simulink model "Main_detection"  (R2015a)
settings: Solver=ode3  StartTime=0.0  StopTime=15  RelTol=1e-3
libraries: legoev3lib x6, simulink x1
settings Model: SimulationMode=external  CovMetricSettings=dwe  CovHtmlReporting=off  covSaveCumulativeToWorkspaceVar=off  CovSaveSingleToWorkspaceVar=off  CovExternalEMLEnable=on  ExtModeTrigDuration=2  Creator=karanverma  LastModifiedBy=karanverma
settings SolverCC: PositivePriorityOrder=on
settings DataIOCC: LimitDataPoints=off  SaveFormat=Dataset
settings OptimizationCC: MaxStackSize=64
settings DebuggingCC: ParameterTunabilityLossMsg=error  SFUnexpectedBacktrackingDiag=error  SFNoUnconditionalDefaultTransitionDiag=error
settings HardwareCC: ProdLargestAtomicInteger=Long  ProdLargestAtomicFloat=Float  ProdIntDivRoundTo=Zero  ProdEndianess=LittleEndian  ProdHWDeviceType=ARM Compatible->ARM 9
settings ModelReferenceCC: PropagateSignalLabelsOutOfModel=on
settings RTWCC: SystemTargetFile=ert.tlc  TLCOptions="-aInlineSetEventsForThisBaseRateFcn=TLC_FALSE -aSuppressMultiTaskScheduler=TLC_FALSE  -aRateBasedStepFcn=0"  TemplateMakefile=ert_default_tmf  Description=Embedded Coder  GenerateReport=on  Toolchain=Sourcery G++ Lite v2009q3  LaunchReport=on
settings CodeAppCC: ForceParamTrailComments=on  OperatorAnnotations=on  MATLABSourceComments=on
settings ERTTargetCC: GenerateSampleERTMain=off  ParMdlRefBuildCompliant=on  CompOptLevelCompliant=on  ConcurrentExecutionCompliant=on  ERTFirstTimeCompliant=on  ERTCustomFileBanners=off  SupportNonInlinedSFcns=on  CPPClassGenCompliant=on  InlinedParameterPlacement=Hierarchical  ConvertIfToSwitch=on  SuppressUnreachableDefaultCases=on

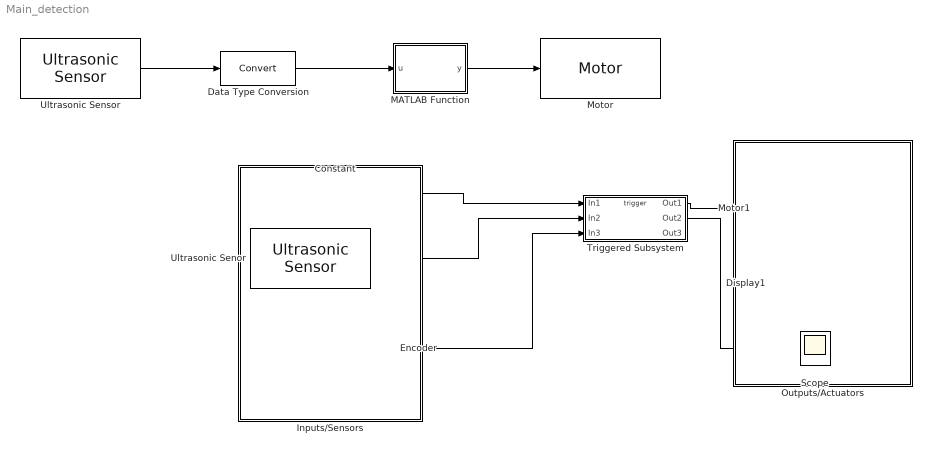
== system Main_detection ==
  Constant : Constant  Value=20
  Data Type Conversion : DataTypeConversion
  Display1 : Display
  Encoder : legoev3lib/Encoder  portNumber=A  opMode=No reset  sampleTime=0.01
  Inputs/Sensors : Subsystem
  MATLAB Function : MATLAB Function  TreatAsAtomicUnit=on
      settings: PermitHierarchicalResolution=ParametersOnly
  Motor : legoev3lib/Motor  sportNumber=A  sstopAction=Brake
  Motor1 : legoev3lib/Motor  sportNumber=A  sstopAction=Brake
  Outputs/Actuators : Subsystem
  Scope : Scope
      settings: TimeRange=auto  MaxDataPoints=5000  SaveName=acqData1  YMin=-90  YMax=80  SampleTime=-1
  Triggered Subsystem : Subsystem  TreatAsAtomicUnit=on
  Ultrasonic Senor : legoev3lib/Ultrasonic Sensor  PortNumber=1  sampleTime=0.01
  Ultrasonic Sensor : legoev3lib/Ultrasonic Sensor  PortNumber=1  sampleTime=0.1
  wires:
  MATLAB Function/1(y) -> Motor/1
  Ultrasonic Sensor/1 -> Data Type Conversion/1
  Data Type Conversion/1 -> MATLAB Function/1(u)
  Constant/1 -> Triggered Subsystem/1(In1)
  Ultrasonic Senor/1 -> Triggered Subsystem/2(In2)
  Encoder/1 -> Triggered Subsystem/3(In3)
  Triggered Subsystem/2(Out2) -> Scope/1
  Triggered Subsystem/1(Out1) -> Motor1/1

== system Main_detection/Inputs//Sensors ==

== system Main_detection/Outputs//Actuators ==

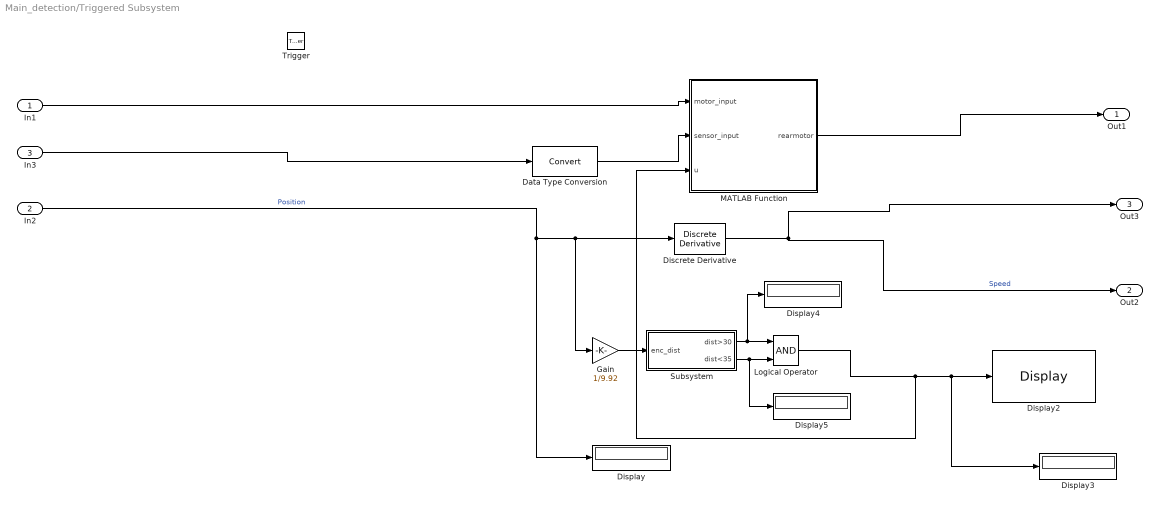
== system Main_detection/Triggered Subsystem ==
  In1 : Inport
  In2 : Inport  Port=2
  In3 : Inport  Port=3
  Trigger : TriggerPort  TriggerType=function-call
  Data Type Conversion : DataTypeConversion
  Discrete Derivative : simulink/Discrete/Discrete Derivative  gainval=1.0  ICPrevScaledInput=800  InputProcessing=Inherited  OutMin=[]  OutMax=[]  OutDataTypeStr=double  OutputDataTypeScalingMode=double  OutDataType=fixdt(1, 16)  OutScaling=2^-10  DoSatur=off
  Display{,3..5} (4 alike) : Display
  Display2 : legoev3lib/Display  slcdStr=Obj_Det  slcdLine=1  slcdFormat=Decimal
  Gain : Gain  Gain=1/9.92
  Logical Operator : Logic  AllPortsSameDT=off  OutDataTypeStr=boolean
  MATLAB Function : MATLAB Function  TreatAsAtomicUnit=on
      settings: PermitHierarchicalResolution=ParametersOnly
  Subsystem : Subsystem
  Out1 : Outport
  Out2 : Outport  Port=2
  Out3 : Outport  Port=3
  wires:
  Data Type Conversion/1 -> MATLAB Function/2(sensor_input)
  MATLAB Function/1(rearmotor) -> Out1/1
  In2/1 -> Gain/1, Discrete Derivative/1, Display/1  "Position"
  In3/1 -> Data Type Conversion/1
  In1/1 -> MATLAB Function/1(motor_input)
  Discrete Derivative/1 -> Out3/1, Out2/1  "Speed"
  Gain/1 -> Subsystem/1(enc_dist)
  Subsystem/1(dist>30) -> Display4/1, Logical Operator/1
  Subsystem/2(dist<35) -> Display5/1, Logical Operator/2
  Logical Operator/1 -> MATLAB Function/3(u), Display3/1, Display2/1

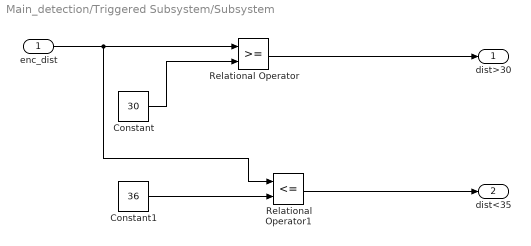
== system Main_detection/Triggered Subsystem/Subsystem ==
  enc_dist : Inport
  Constant : Constant  Value=30
  Constant1 : Constant  Value=36
  Relational Operator : RelationalOperator  OutDataTypeStr=boolean
  Relational Operator1 : RelationalOperator  Operator=<=  OutDataTypeStr=boolean
  dist>30 : Outport
  dist<35 : Outport  Port=2
  wires:
  enc_dist/1 -> Relational Operator1/1, Relational Operator/1
  Constant/1 -> Relational Operator/2
  Constant1/1 -> Relational Operator1/2
  Relational Operator/1 -> dist>30/1
  Relational Operator1/1 -> dist<35/1

== matlab function Main_detection/Triggered Subsystem/MATLAB Function ==
  data: motor_input input; sensor_input input; rearmotor output; u input
function rearmotor = fcn(motor_input,sensor_input,u)
%#codegen
if(sensor_input>4)&&(sensor_input<=20)&& (u==1)
    rearmotor=motor_input;
%elseif(sensor_input>20)&&(sensor_input<=35)
 %   rearmotor=motor_input;
else
    rearmotor=0;
end
end

== matlab function Main_detection/MATLAB Function ==
  data: u input; y output
function y = fcn(u)

if(u<4)&&(u>=40) 
    y = 20;
    
    
end
end
